simulink model "asbhl20_FCSApp"  (R2016b)
settings: Solver=FixedStepDiscrete  StartTime=0.0  StopTime=10.0  FixedStep=1/60  RelTol=1e-3
values from neighbouring files (symbols this model uses):
  Kalpha_1 = [0.0675525766417 0.0670941520285 0.105277724217 0.0705938909254 0.0692391670282 0.0682506457138 0.0672739862702 0.0668102273189]    [asbhl20_FCSAppData.mat]
  Kbeta_1 = [-0.0493656538568 -0.0419788515038 -0.0374619432887 -0.0381850673629 -0.0395050518916 -0.0416555062349 -0.0442775778109 -0.0483706672557]    [asbhl20_FCSAppData.mat]
  Kp_1 = [60.2253428509 52.7939261692 51.6224369342 53.1835874806 55.9559014793 59.5393657693 64.8225348547 75.6927037235]    [asbhl20_FCSAppData.mat]
  Kphi_1 = [5.15511075546 5.17463543618 5.19891345689 5.21223828381 5.13966398998 5.1414152167 5.20955736592 5.29359350801]    [asbhl20_FCSAppData.mat]
  Kq_1 = [-190.665384898 -180.322553126 -174.03272401 -173.493656781 -180.877109643 -197.917252796 -228.270830002 -278.51108854]    [asbhl20_FCSAppData.mat]
  Kr_1 = [-714.366713062 -1002.72404317 -1151.4783324 -1152.96908365 -1070.59786805 -1009.08046077 -1000.48966647 -1058.93322007]    [asbhl20_FCSAppData.mat]
  qbar0 = 10722.8924586    [asbhl20_FCSAppData.mat]
  U_trim_matrix = [-23.7683817467 -4.33440943636 4.43733647183 -22.1955716586 4.52075664841 21.6532360323 -20.4783849922 6.34956743865 19.7065472455 -22.2662158495 5.88613316784 30.8883374276 ... (120 elements, 3x8x5)]    [asbhl20_FCSAppData.mat]
undefined symbols (not defined in the file or in its folder): Tc
libraries: discretizing x4, aerolibconvert2 x3
Description:
  | HL-20 Flight Control System module
settings Model: FPTRunName=Active  ExtModeAutoUpdateStatusClock=off  Creator=The MathWorks, Inc.  LastModifiedBy=The MathWorks, Inc.
settings DataIOCC: SaveFormat=Array  SaveOutput=off  SaveTime=off
settings OptimizationCC: BlockReduction=off  DefaultParameterBehavior=Inlined  OptimizeBlockIOStorage=off  BufferReuse=off  GlobalBufferReuse=off  ExpressionFolding=off  ExpressionDepthLimit=2147483647  LocalBlockOutputs=off  InitFltsAndDblsToZero=on  LifeSpan=inf
settings DebuggingCC: SaveWithParameterizedLinksMsg=none  SolverPrmCheckMsg=warning  MultiTaskCondExecSysMsg=none  FcnCallInpInsideContextMsg=warning  UniqueDataStoreMsg=error  AllowSymbolicDim=off  StateNameClashWarn=warning  StrictBusMsg=ErrorOnBusTreatedAsVector  SFUnexpectedBacktrackingDiag=warning  SFNoUnconditionalDefaultTransitionDiag=warning  SFExecutionAtInitializationDiag=none
settings HardwareCC: ProdBitPerPointer=32  ProdBitPerSizeT=32  ProdBitPerPtrDiffT=32  ProdLargestAtomicFloat=None  ProdIntDivRoundTo=Undefined  ProdEndianess=Unspecified  ProdWordSize=32  ProdHWDeviceType=32-bit Generic
settings ModelReferenceCC: UpdateModelReferenceTargets=AssumeUpToDate  CheckModelReferenceTargetMessage=none  ModelReferencePassRootInputsByReference=off  PropagateSignalLabelsOutOfModel=off
settings CodeAppCC: MaxIdLength=63
settings GRTTargetCC: TargetFcnLib=ansi_tfl_tmw.mat  TargetLangStandard=C89/C90 (ANSI)  GeneratePreprocessorConditionals=Disable all  CombineOutputUpdateFcns=off  GRTInterface=on
settings ConfigComp: CovMetricSettings=dw  CovHtmlReporting=on  CovSaveCumulativeToWorkspaceVar=on  CovSaveSingleToWorkspaceVar=on  CovExternalEMLEnable=off  CovSFcnEnable=off

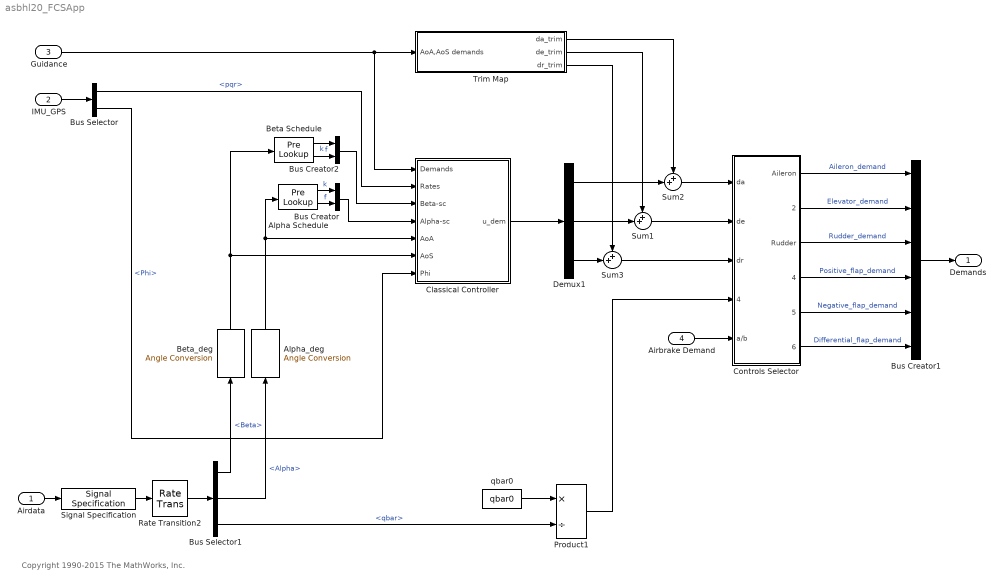
== system asbhl20_FCSApp ==
  note: Copyright 1990-2015 The MathWorks, Inc.
  Airdata : Inport  OutDataTypeStr=Bus: AirDataBus
  IMU_GPS : Inport  Port=2  OutDataTypeStr=Bus: FCSSensorBus
  Guidance : Inport  Port=3  PortDimensions=3
  Airbrake Demand : Inport  Port=4
  Alpha Schedule : PreLookup  BreakpointsData=a_vec  BeginIndexSearchUsingPreviousIndexResult=on  ExtrapMethod=Linear
  Alpha_deg : aerolibconvert2/Angle Conversion  IU=rad  OU=deg
  Beta Schedule : PreLookup  BreakpointsData=b_vec  BeginIndexSearchUsingPreviousIndexResult=on  ExtrapMethod=Linear
  Beta_deg : aerolibconvert2/Angle Conversion  IU=rad  OU=deg
  Bus Creator : BusCreator  Inputs=2
  Bus Creator1 : BusCreator  Inputs=6  OutDataTypeStr=Bus: FCSCmdBus  NonVirtualBus=on
  Bus Creator2 : BusCreator  Inputs=2
  Bus Selector : BusSelector  OutputSignals=pqr,Phi
  Bus Selector1 : BusSelector  OutputSignals=Beta,Alpha,qbar
  Classical Controller : Subsystem
  Controls Selector : Subsystem
  Demux1 : Demux  Outputs=3
  Product1 : Product  Inputs=*/  SaturateOnIntegerOverflow=on  InputSameDT=on  OutDataTypeStr=Inherit: Same as first input
  Rate Transition2 : RateTransition  OutPortSampleTime=Tf
  Signal Specification : SignalSpecification  SampleTime=Tc
  Sum1 : Sum  Inputs=++|  SaturateOnIntegerOverflow=on  InputSameDT=on  OutDataTypeStr=Inherit: Same as first input
  Sum2 : Sum  Inputs=++|  SaturateOnIntegerOverflow=on  InputSameDT=on  OutDataTypeStr=Inherit: Same as first input
  Sum3 : Sum  Inputs=++|  SaturateOnIntegerOverflow=on  InputSameDT=on  OutDataTypeStr=Inherit: Same as first input
  Trim Map : Subsystem
  qbar0 : Constant  Value=qbar0  OutDataTypeStr=Inherit: Inherit via back propagation  SampleTime=Tc
  Demands : Outport  OutDataTypeStr=Bus: FCSCmdBus
  wires:
  qbar0/1 -> Product1/1
  Bus Selector1/2 -> Alpha_deg/1  "<Alpha>"
  Bus Selector1/1 -> Beta_deg/1  "<Beta>"
  Bus Selector1/3 -> Product1/2  "<qbar>"
  Bus Creator1/1 -> Demands/1
  Bus Creator/1 -> Classical Controller/4(Alpha-sc)
  Bus Creator2/1 -> Classical Controller/3(Beta-sc)
  Bus Selector/1 -> Classical Controller/2(Rates)  "<pqr>"
  Guidance/1 -> Classical Controller/1(Demands), Trim Map/1(AoA,AoS demands)
  Alpha_deg/1 -> Classical Controller/5(AoA), Alpha Schedule/1
  Controls Selector/1(Aileron) -> Bus Creator1/1  "Aileron_demand"
  Controls Selector/2(Elevator) -> Bus Creator1/2  "Elevator_demand"
  Controls Selector/3(Rudder) -> Bus Creator1/3  "Rudder_demand"
  Controls Selector/4(Flap(pos)) -> Bus Creator1/4  "Positive_flap_demand"
  Controls Selector/5(Flap(neg)) -> Bus Creator1/5  "Negative_flap_demand"
  Controls Selector/6(Flap(diff)) -> Bus Creator1/6  "Differential_flap_demand"
  Beta_deg/1 -> Classical Controller/6(AoS), Beta Schedule/1
  Product1/1 -> Controls Selector/4(qbar_inv)
  Sum2/1 -> Controls Selector/1(da)
  Trim Map/1(da_trim) -> Sum2/1
  Sum1/1 -> Controls Selector/2(de)
  Sum3/1 -> Controls Selector/3(dr)
  Trim Map/2(de_trim) -> Sum1/1
  Trim Map/3(dr_trim) -> Sum3/1
  Demux1/2 -> Sum1/2
  Demux1/3 -> Sum3/2
  Demux1/1 -> Sum2/2
  Classical Controller/1(u_dem) -> Demux1/1
  IMU_GPS/1 -> Bus Selector/1
  Bus Selector/2 -> Classical Controller/7(Phi)  "<Phi>"
  Airdata/1 -> Signal Specification/1
  Airbrake Demand/1 -> Controls Selector/5(a/b)
  Signal Specification/1 -> Rate Transition2/1
  Rate Transition2/1 -> Bus Selector1/1
  Alpha Schedule/1 -> Bus Creator/1  "k"
  Alpha Schedule/2 -> Bus Creator/2  "f"
  Beta Schedule/1 -> Bus Creator2/1  "k"
  Beta Schedule/2 -> Bus Creator2/2  "f"

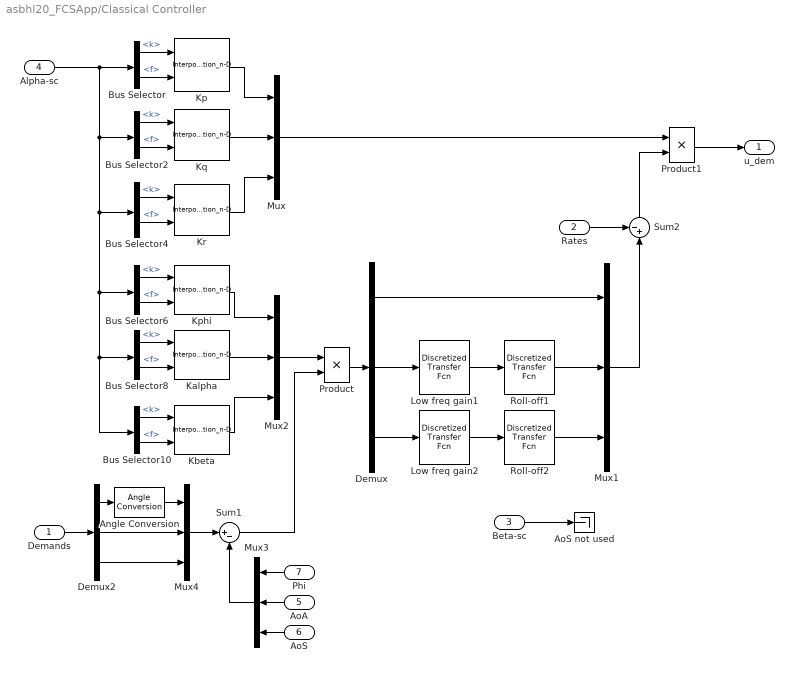
== system asbhl20_FCSApp/Classical Controller ==
  Demands : Inport  PortDimensions=3
  Rates : Inport  Port=2  PortDimensions=3
  Beta-sc : Inport  Port=3
  Alpha-sc : Inport  Port=4
  AoA : Inport  Port=5  PortDimensions=1
  AoS : Inport  Port=6  PortDimensions=1
  Phi : Inport  Port=7  PortDimensions=1
  Angle Conversion : aerolibconvert2/Angle Conversion  IU=deg  OU=rad
  AoS not used : Terminator
  Bus Selector{,2,4,6,8,10} (6 alike) : BusSelector  OutputSignals=k,f
  Demux : Demux  Outputs=3
  Demux2 : Demux  Outputs=3
  Kalpha : Interpolation_n-D  NumberOfTableDimensions=1  Table=Kalpha_1  RemoveProtectionIndex=on
      settings: InputPortMap=u0,u1
  Kbeta : Interpolation_n-D  NumberOfTableDimensions=1  Table=Kbeta_1  RemoveProtectionIndex=on
      settings: InputPortMap=u0,u1
  Kp : Interpolation_n-D  NumberOfTableDimensions=1  Table=Kp_1  RemoveProtectionIndex=on
      settings: InputPortMap=u0,u1
  Kphi : Interpolation_n-D  NumberOfTableDimensions=1  Table=Kphi_1  RemoveProtectionIndex=on
      settings: InputPortMap=u0,u1
  Kq : Interpolation_n-D  NumberOfTableDimensions=1  Table=Kq_1  RemoveProtectionIndex=on
      settings: InputPortMap=u0,u1
  Kr : Interpolation_n-D  NumberOfTableDimensions=1  Table=Kr_1  RemoveProtectionIndex=on
      settings: InputPortMap=u0,u1
  Low freq gain1 : discretizing/Discretized Transfer Fcn  Numerator=[1, 2]  Denominator=[1, 0]  AbsTol=auto  SampleTime=Tc  method=zoh  Wc=1
  Low freq gain2 : discretizing/Discretized Transfer Fcn  Numerator=[1, 0.5]  Denominator=[1, 0]  AbsTol=auto  SampleTime=Tc  method=zoh  Wc=1
  Mux{,1,3..4} (4 alike) : Mux  Inputs=[1,1,1]
  Mux2 : Mux  Inputs=3
  Product : Product  SaturateOnIntegerOverflow=on  InputSameDT=on  OutDataTypeStr=Inherit: Same as first input
  Product1 : Product  SaturateOnIntegerOverflow=on  InputSameDT=on  OutDataTypeStr=Inherit: Same as first input
  Roll-off1 : discretizing/Discretized Transfer Fcn  Numerator=10  Denominator=[1, 10]  AbsTol=auto  SampleTime=Tc  method=zoh  Wc=1
  Roll-off2 : discretizing/Discretized Transfer Fcn  Numerator=10  Denominator=[1, 10]  AbsTol=auto  SampleTime=Tc  method=zoh  Wc=1
  Sum1 : Sum  Inputs=|+-  SaturateOnIntegerOverflow=on  InputSameDT=on  OutDataTypeStr=Inherit: Same as first input
  Sum2 : Sum  Inputs=-+|  SaturateOnIntegerOverflow=on  InputSameDT=on  OutDataTypeStr=Inherit: Same as first input
  u_dem : Outport  InitialOutput=[0 0 0]
  wires:
  Alpha-sc/1 -> Bus Selector10/1, Bus Selector8/1, Bus Selector6/1, Bus Selector4/1, Bus Selector2/1, Bus Selector/1
  Bus Selector8/2 -> Kalpha/2  "<f>"
  Bus Selector10/2 -> Kbeta/2  "<f>"
  Bus Selector10/1 -> Kbeta/1  "<k>"
  Bus Selector8/1 -> Kalpha/1  "<k>"
  Bus Selector6/2 -> Kphi/2  "<f>"
  Bus Selector6/1 -> Kphi/1  "<k>"
  Bus Selector4/2 -> Kr/2  "<f>"
  Bus Selector4/1 -> Kr/1  "<k>"
  Bus Selector2/2 -> Kq/2  "<f>"
  Bus Selector2/1 -> Kq/1  "<k>"
  Bus Selector/2 -> Kp/2  "<f>"
  Bus Selector/1 -> Kp/1  "<k>"
  Kq/1 -> Mux/2
  Kp/1 -> Mux/1
  Kr/1 -> Mux/3
  Mux3/1 -> Sum1/2
  Phi/1 -> Mux3/1
  AoA/1 -> Mux3/2
  AoS/1 -> Mux3/3
  Mux2/1 -> Product/1
  Sum1/1 -> Product/2
  Product/1 -> Demux/1
  Rates/1 -> Sum2/1
  Mux/1 -> Product1/1
  Sum2/1 -> Product1/2
  Mux1/1 -> Sum2/2
  Kalpha/1 -> Mux2/2
  Kbeta/1 -> Mux2/3
  Kphi/1 -> Mux2/1
  Demands/1 -> Demux2/1
  Demux2/1 -> Angle Conversion/1
  Angle Conversion/1 -> Mux4/1
  Demux2/2 -> Mux4/2
  Demux2/3 -> Mux4/3
  Mux4/1 -> Sum1/1
  Product1/1 -> u_dem/1
  Beta-sc/1 -> AoS not used/1
  Demux/1 -> Mux1/1
  Roll-off2/1 -> Mux1/3
  Roll-off1/1 -> Mux1/2
  Demux/3 -> Low freq gain2/1
  Demux/2 -> Low freq gain1/1
  Low freq gain1/1 -> Roll-off1/1
  Low freq gain2/1 -> Roll-off2/1

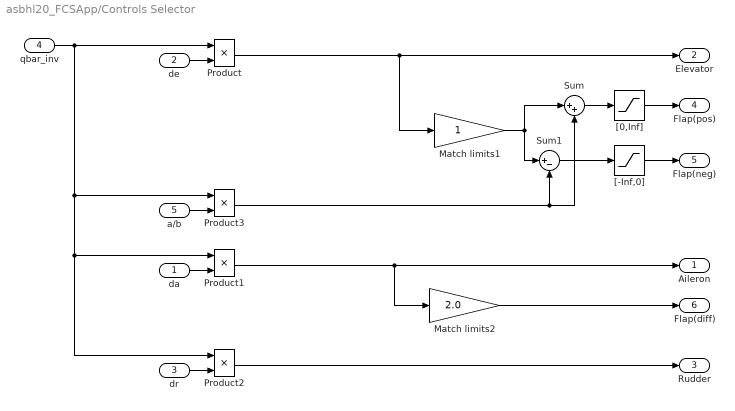
== system asbhl20_FCSApp/Controls Selector ==
  da : Inport
  de : Inport  Port=2
  dr : Inport  Port=3
  qbar_inv : Inport  Port=4
  a/b : Inport  Port=5
  Match limits1 : Gain  SaturateOnIntegerOverflow=on  OutDataTypeStr=Inherit: Same as input  ParamDataTypeStr=Inherit: Same as input
  Match limits2 : Gain  Gain=2.0  SaturateOnIntegerOverflow=on  OutDataTypeStr=Inherit: Same as input  ParamDataTypeStr=Inherit: Same as input
  Product{,1..3} (4 alike) : Product  SaturateOnIntegerOverflow=on  InputSameDT=on  OutDataTypeStr=Inherit: Same as first input
  Sum : Sum  Inputs=|++  SaturateOnIntegerOverflow=on  InputSameDT=on  OutDataTypeStr=Inherit: Same as first input
  Sum1 : Sum  Inputs=|+-  SaturateOnIntegerOverflow=on  InputSameDT=on  OutDataTypeStr=Inherit: Same as first input
  "[-Inf,0]" : Saturate  UpperLimit=0  LowerLimit=-Inf
  "[0,Inf]" : Saturate  UpperLimit=Inf  LowerLimit=0
  Aileron : Outport
  Elevator : Outport  Port=2
  Rudder : Outport  Port=3
  Flap(pos) : Outport  Port=4
  Flap(neg) : Outport  Port=5
  Flap(diff) : Outport  Port=6
  wires:
  qbar_inv/1 -> Product/1, Product2/1, Product1/1, Product3/1
  de/1 -> Product/2
  Product2/1 -> Rudder/1
  dr/1 -> Product2/2
  da/1 -> Product1/2
  Product1/1 -> Match limits2/1, Aileron/1
  Product/1 -> Elevator/1, Match limits1/1
  Match limits1/1 -> Sum/1, Sum1/1
  "[-Inf,0]"/1 -> Flap(neg)/1
  "[0,Inf]"/1 -> Flap(pos)/1
  Match limits2/1 -> Flap(diff)/1
  a/b/1 -> Product3/2
  Sum/1 -> "[0,Inf]"/1
  Sum1/1 -> "[-Inf,0]"/1
  Product3/1 -> Sum1/2, Sum/2

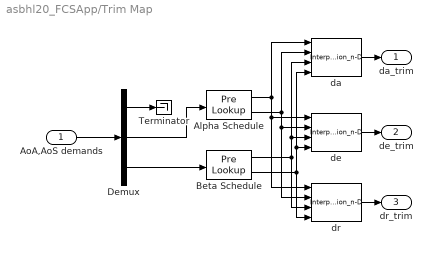
== system asbhl20_FCSApp/Trim Map ==
  AoA,AoS demands : Inport
  Alpha Schedule : PreLookup  BreakpointsData=a_vec  BeginIndexSearchUsingPreviousIndexResult=on  ExtrapMethod=Linear
  Beta Schedule : PreLookup  BreakpointsData=b_vec  BeginIndexSearchUsingPreviousIndexResult=on  ExtrapMethod=Linear
  Demux : Demux  Outputs=3
  Terminator : Terminator
  da : Interpolation_n-D  Table=squeeze(U_trim_matrix(1,:,:))  RemoveProtectionIndex=on
  de : Interpolation_n-D  Table=squeeze(U_trim_matrix(2,:,:))  RemoveProtectionIndex=on
  dr : Interpolation_n-D  Table=squeeze(U_trim_matrix(3,:,:))  RemoveProtectionIndex=on
  da_trim : Outport
  de_trim : Outport  Port=2
  dr_trim : Outport  Port=3
  wires:
  Beta Schedule/2 -> dr/4, de/4, da/4
  Alpha Schedule/2 -> dr/2, de/2, da/2
  Alpha Schedule/1 -> da/1, dr/1, de/1
  Beta Schedule/1 -> dr/3, de/3, da/3
  AoA,AoS demands/1 -> Demux/1
  Demux/2 -> Alpha Schedule/1
  Demux/3 -> Beta Schedule/1
  Demux/1 -> Terminator/1
  da/1 -> da_trim/1
  de/1 -> de_trim/1
  dr/1 -> dr_trim/1
